simulink library "lib_Convection_LamIncompFlatPlateBL"  (R2015a)
settings: Solver=ode45  StartTime=0.0  StopTime=10.0  RelTol=1e-3
libraries: simulink x1
settings Model: Creator=jlkratz  LastModifiedBy=jlkratz

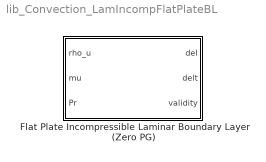
== system lib_Convection_LamIncompFlatPlateBL ==
  Flat Plate Incompressible Laminar Boundary Layer (Zero PG) : Subsystem  mask(TSAT: Flat Plate Incompressible Laminar Boundary Layer (Zero PG)){Retr_M=500000, x_M=1}
      mask prompts: Retr_M "Retr_M - Transition Reynolds number"; x_M "x_M - Local position from the leading edge"
      mask help: This block approximates the boundary layer and thermal boundary layer thicknesses of incompressible laminar flow over a flat plate with a pressure gradient of 0.
      mask Help: web(which('Convection_TSAT_LamIncompFlatPlateBL.html'),'-helpbrowser')
      mask DialogControl Container3 Prompt: Parameters

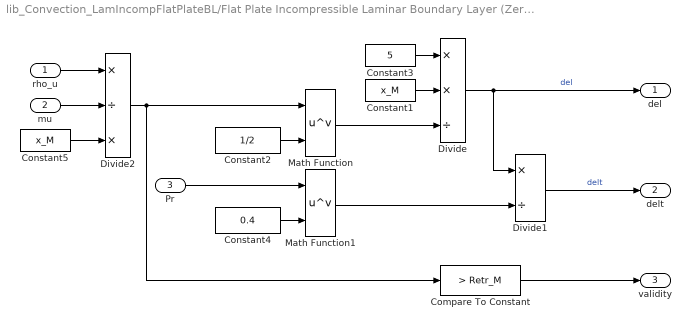
== system lib_Convection_LamIncompFlatPlateBL/Flat Plate Incompressible Laminar Boundary Layer (Zero PG) ==
  rho_u : Inport
  mu : Inport  Port=2
  Pr : Inport  Port=3
  Compare To Constant : simulink/Logic and Bit Operations/Compare To Constant  relop=>  const=Retr_M  OutDataTypeStr=boolean
  Constant1 : Constant  Value=x_M
  Constant2 : Constant  Value=1/2
  Constant3 : Constant  Value=5
  Constant4 : Constant  Value=0.4
  Constant5 : Constant  Value=x_M
  Divide : Product  Inputs=**/
  Divide1 : Product  Inputs=*/
  Divide2 : Product  Inputs=*/*
  Math Function : Math  Operator=pow  SaturateOnIntegerOverflow=on
  Math Function1 : Math  Operator=pow  SaturateOnIntegerOverflow=on
  del : Outport
  delt : Outport  Port=2
  validity : Outport  Port=3
  wires:
  Compare To Constant/1 -> validity/1
  Math Function1/1 -> Divide1/2
  Divide/1 -> Divide1/1, del/1  "del"
  Constant4/1 -> Math Function1/2
  Math Function/1 -> Divide/3
  Pr/1 -> Math Function1/1
  Divide1/1 -> delt/1  "delt"
  Constant2/1 -> Math Function/2
  Constant3/1 -> Divide/1
  Constant1/1 -> Divide/2
  rho_u/1 -> Divide2/1
  Constant5/1 -> Divide2/3
  mu/1 -> Divide2/2
  Divide2/1 -> Compare To Constant/1, Math Function/1
